simulink model "pulseCounter"  (R2020b)
settings: Solver=VariableStepAuto  StartTime=0.0  StopTime=10.0  RelTol=1e-3
libraries: simulink x1
settings Model: Creator=Balazs  LastModifiedBy=Balazs

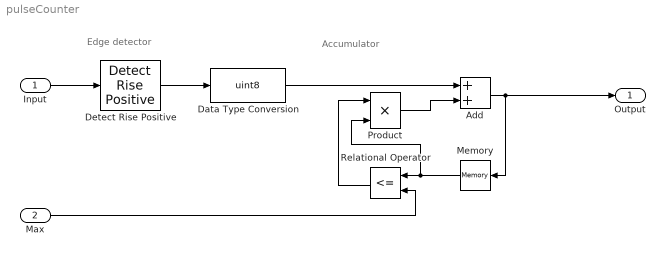
== system pulseCounter ==
  note: Accumulator
  note: Edge detector
  Input : Inport  OutDataTypeStr=boolean
  Max : Inport  Port=2  OutDataTypeStr=uint8
  Add : Sum
  Data Type Conversion : DataTypeConversion  OutDataTypeStr=uint8
  Detect Rise Positive : simulink/Logic and Bit Operations/Detect Rise Positive  vinit=0  OutDataTypeStr=boolean
  Memory : Memory
  Product : Product  OutDataTypeStr=uint8
  Relational Operator : RelationalOperator  Operator=<=  OutDataTypeStr=boolean  RndMeth=Simplest
  Output : Outport  OutDataTypeStr=uint8
  wires:
  Input/1 -> Detect Rise Positive/1
  Add/1 -> Memory/1, Output/1
  Detect Rise Positive/1 -> Data Type Conversion/1
  Data Type Conversion/1 -> Add/1
  Memory/1 -> Relational Operator/1, Product/2
  Product/1 -> Add/2
  Relational Operator/1 -> Product/1
  Max/1 -> Relational Operator/2
